simulink model "VCO"  (R2019b)
settings: Solver=VariableStepAuto  StartTime=0.0  StopTime=10.0  RelTol=1e-3
model workspace (MAT data in the model file):
  Frequency_10 = 32099999.9999
  LockTime_10 = 9.96884735202e-07
  VcoParamResultTable = [nan nan]
  frequencyVector = [25097868.3513 nan nan nan nan nan nan nan nan nan]
  kvcoVector = [nan nan nan nan nan nan nan nan nan]
  quiescentFreq = nan
  vctrlVector = [1 1.44 1.89 2.33 2.78 3.22 3.67 4.11 4.56 5]
libraries: msbPllMeasurements x2, msbPllArchitectures x1, msbPllFoundation x1
settings Model: OrderedModelArguments=off  Creator=lfbarrag  LastModifiedBy=lfbarrag

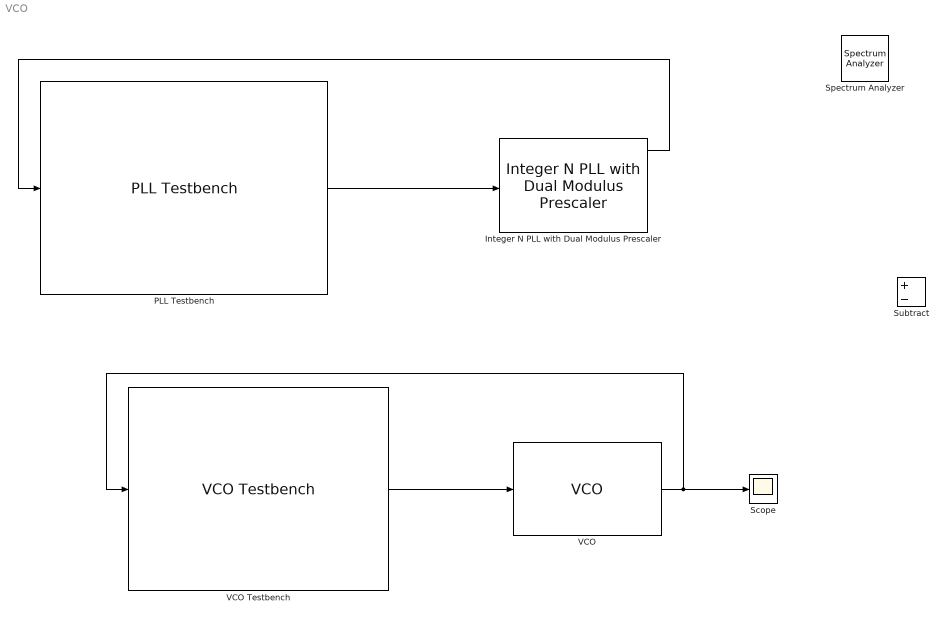
== system VCO ==
  Integer N PLL with Dual Modulus Prescaler : msbPllArchitectures/Integer N PLL with Dual Modulus Prescaler  DeadbandCompensation=40e-12  EnableImpairments=off  DefaultOrAdvanced=Default  MaxFreqInterest=10e9  RiseFallTime=3e-11  PropDelay=50e-12  OutputCurrent=4e-3  InputThreshold=5  EnableCurrentImpairments=off  CurrentImbalance=1e-7  LeakageCurrent=1e-8  EnableTimingImpairments=off  DefaultOrAdvancedCp=Default  MaxFreqInterestCp=10e9  RiseFallUp=50e-12  PropDelayUp=60e-12  RiseFallDown=20e-12  PropDelayDown=40e-12  SpecifyUsing=Voltage sensitivity  Kvco=1.4  ControlVoltage=[-5 0 5]  OutputFrequency=[2e9 2.5e9 3e9]  MaxKvco=1.4  Fo=32.1e6  Amplitude=1  AddPhaseNoise=off  Foffset=[100 200 300 400 1000 2000 5000 100000 250000]  PhaseNoise=[-35.8 -65 -70 -72.9 -83.4 -89 -90.1 -96.5 -111.6]  ProgramCounter=100  PrescalerDivider=8  SwallowCounter=9  EffectiveDividerValue=0  Nmin=809  CompSelectionMethod=Manual  Fc=1e6  Phi=45  FilterType="3rd  order passive"  C1=12e-9  C2=80e-9  C3=220e-9  C4=1e-12  R2=62e3  R3=1e3  R4=12e3  LfEnableImpairments=off  Temperature=30  pfd_up_dn=off  cp_out=on  lf_out=on  ps_out=on  ol_opt=on  cl_opt=on  ExtraBuffer=off  NBufferFilter=1000  NBuffer=10
      settings: SourceProductName=Mixed-Signal Blockset  SourceProductBaseCode=AM
  PLL Testbench : msbPllMeasurements/PLL Testbench  InputAmplitude=1  ClkFreq=10e6  FrequencyMeasureOption=on  CurrentFrequency=0  LockTimeOption=on  ExpectedFreq=32.1e6  FreqErrorTol=5e4  CurrentLockTime=0  PhaseNoiseOption=off  SampleRate=4*32.1e6  ResBandwidth=25e3  SpectralAverages=1  HoldOffTime=0  PhaseNoiseFreqOffset=[300e3 1e5 1e6]  OpenSpectrum=on  ExtraBuffer=off  NBuffer=10  PowerVector=0  FrequencyVector=0  TargetFreq=2.1e9  TargetLockTime=3e-6  TargetPhaseNoiseVector=[-85,-125,-180]
      settings: SourceProductName=Mixed-Signal Blockset  SourceProductBaseCode=AM  SignalType=Square
  Scope : Scope
  Spectrum Analyzer : SpectrumAnalyzer
  Subtract : Sum  Inputs=+-
  VCO : msbPllFoundation/VCO  SpecifyUsing=Output frequency vs. control voltage  Kvco=1.4e0  Fo=2.5e9  ControlVoltage=[1 5]  OutputFrequency=[25e6 35e6]  Amplitude=1  ExtraBuffer=off  NBuffer=10  AddPhaseNoise=off  Foffset=[100 200 300 400 1000 2000 5000 100000 250000]  PhaseNoise=[-35.8 -65 -70 -72.9 -83.4 -89 -90.1 -96.5 -111.6]  MaxKvco=2500000
      settings: SourceProductName=Mixed-Signal Blockset  SourceProductBaseCode=AM
  VCO Testbench : msbPllMeasurements/VCO Testbench  MeasureOptions=Kvco and Fo  ControlVoltage=5  ControlVoltageRange=[1 5]  ControlVoltageVector=[1.00, 1.44, 1.89, 2.33, 2.78, 3.22, 3.67, 4.11, 4.56, 5.00]  TsampStair=1  SampleFrequency=4*32.1e6  ResBandwidth=5e4  SpectralAverages=4  ExtraBuffer=off  NBuffer=10  PowerVector=0  FrequencyVector=0  HoldOffTime=1e-3  PhaseNoiseFreqOffset=[30e3 100e3 1e6 3e6 10e6]  PhaseNoiseVector=[-50 -106 -132 -143 -152]
      settings: SourceProductName=Mixed-Signal Blockset  SourceProductBaseCode=AM
  wires:
  VCO Testbench/1 -> VCO/1
  VCO/1 -> Scope/1, VCO Testbench/1
  PLL Testbench/1 -> Integer N PLL with Dual Modulus Prescaler/1
  Integer N PLL with Dual Modulus Prescaler/1 -> PLL Testbench/1
